simulink library "tqr"  (R2021b)
settings: Solver=VariableStepAuto  StartTime=0.0  StopTime=10.0  RelTol=1e-3
undefined symbols (not defined in the file or in its folder): ATQR_AltRDCActiveFEDUInc_X_pct, ATQR_AltRDCActiveFEDUInc_Y_enum, ATQR_AltRDCActiveFEDUTs_X_pct, ATQR_AltRDCActiveFEDUTs_Y_enum, ATQR_AltRDCActiveREDUInc_X_pct, ATQR_AltRDCActiveREDUInc_Y_enum, ATQR_AltRDCActiveREDUTs_X_pct, ATQR_AltRDCActiveREDUTs_Y_enum, ATQR_CreepFEDUTqIncSR_X_rpm, ATQR_CreepFEDUTqIncSR_Y_Nm, ATQR_CreepFEDUTs_X_rpm, ATQR_CreepFEDUTs_Y_Nm, ATQR_EcoTqFrIncGain_X_Nm, ATQR_EcoTqFrIncGain_Y_pct, ATQR_EcoTqRrIncGain_X_Nm, ATQR_EcoTqRrIncGain_Y_pct, ATQR_EL1FEDUTqDecSR_Y_Nm, ATQR_EL1FEDUTqIncSR_X_rpm, ATQR_EL1FEDUTqIncSR_Y_pct, ATQR_EL1FEDUTs_X_rpm, ATQR_EL1FEDUTs_Y_Nm, ATQR_EL1REDUTqDecSR_Y_Nm, ATQR_EL1REDUTs_Y_Nm, ATQR_FEDUEL1RegenTs_X_rpm, ATQR_FEDUTIPOutTs_X_rpm, ATQR_FrNegRateLimitIncN_X_rpm, ATQR_FrNegRateLimitIncN_Y_Nm, ATQR_FrPosRateLimitIncN_X_rpm, ATQR_FrPosRateLimitIncN_Y_Nm, ATQR_FShaftSpdTqLimCoe_X_rpm, ATQR_FTimerTqLimCoe_X_s, ATQR_FTqZeroTransUpBoundN_X_rpm, ATQR_NL1FEDUTqDecSR_Y_Nm, ATQR_NL1FEDUTqIncSR_X_rpm, ATQR_NL1FEDUTqIncSR_Y_pct, ATQR_NL1FEDUTs_X_rpm, ATQR_NL1FEDUTs_Y_Nm, ATQR_NL1REDUTqDecSR_Y_Nm, ATQR_NL1REDUTs_Y_Nm, ATQR_NormalTqFrIncGain_X_Nm, ATQR_NormalTqFrIncGain_Y_pct, ATQR_NormalTqRrIncGain_X_Nm, ATQR_NormalTqRrIncGain_Y_pct, ATQR_RrNegRateLimitIncN_X_rpm, ATQR_RrNegRateLimitIncN_Y_Nm, ATQR_RrPosRateLimitIncN_X_rpm, ATQR_RrPosRateLimitIncN_Y_Nm, ATQR_RShaftSpdTqLimCoe_X_rpm, ATQR_RTimerTqLimCoe_X_s, ATQR_SL1FEDUTqDecSR_Y_Nm, ATQR_SL1FEDUTqIncSR_X_rpm, ATQR_SL1FEDUTqIncSR_Y_pct, ATQR_SL1FEDUTs_X_rpm, ATQR_SL1FEDUTs_Y_Nm, ATQR_SL1REDUTqDecSR_Y_Nm, ATQR_SL1REDUTs_Y_Nm, ATQR_SportTqFrIncGain_X_Nm, ATQR_SportTqFrIncGain_Y_pct, ATQR_SportTqRrIncGain_X_Nm, ATQR_SportTqRrIncGain_Y_pct ... (+269)
libraries: hcu_lib x15, simulink x13, $bdroot x3
(part 1 of 9)
settings Model: Creator=13615  LastModifiedBy=FVT23118
settings SolverCC: AlgebraicLoopSolver=TrustRegion
settings DataIOCC: SaveFormat=Array  SignalLoggingSaveFormat=ModelDataLogs  ReturnWorkspaceOutputs=off
settings OptimizationCC: BlockReduction=off  BooleanDataType=off
settings DebuggingCC: SaveWithParameterizedLinksMsg=none  UnderspecifiedInitializationDetection=Classic  MergeDetectMultiDrivingBlocksExec=none  SignalResolutionControl=TryResolveAllWithWarning  SFMachineParentedDataDiag=warning
settings HardwareCC: TargetUnknown=on
settings ModelReferenceCC: PropagateSignalLabelsOutOfModel=off
settings ConfigComp: CovMetricSettings=dw  CovSaveCumulativeToWorkspaceVar=on  CovSaveSingleToWorkspaceVar=on

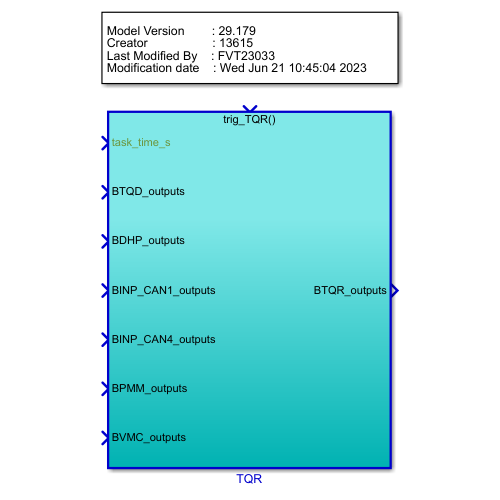
[thumbnail: Simulink's stored preview of the top-level diagram]
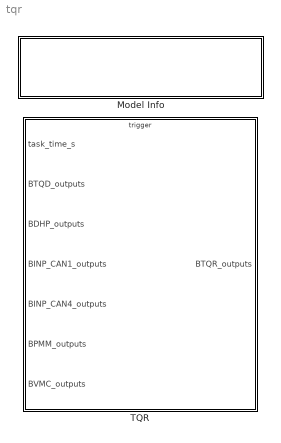
== system tqr ==
  Model Info : Subsystem  LoadFcn=slcm LoadBlock;  InitFcn=slcm('UpdateAllCMBlocksInThisModelInit')  mask(CMBlock){InitialSaveTempField=, InitialBlockCM=None, BlockCM=None, Frame=on, SaveTempField=, DisplayStringWithTags=|, MaskDisplayString=Model Version        : 29.417\nCreator                   : 13615\nLast Modified By    : FVT23118\nModification date    : Thu Aug 29 10:52:14 2024, HorizontalTextAlignment=Left, LeftAlignmentValue=0.02, SourceBlockDiagram=tqr, TagMaxNumber=20, CMTag1=, CMTag2=, CMTag3=, CMTag4=, CMTag5=, CMTag6=, CMTag7=, CMTag8=, CMTag9=, CMTag10=, CMTag11=, CMTag12=, CMTag13=, CMTag14=, CMTag15=, CMTag16=, CMTag17=, CMTag18=, CMTag19=, CMTag20=}
      mask DisplayStringWithTags=|
      | Model Version        : %<ModelVersion>
      | Creator                   : %<Creator>
      | Last Modified By    : %<LastModifiedBy>
      | Modification date    : %<LastModificationDate>
      mask help: This block allows revision control information to be displayed within the model.
      settings: CopyFcn=slcm CopyBlock;  DeleteFcn=slcm Cancel;  PostSaveFcn=slcm('UpdateAllCMBlocksInThisModel')  NameChangeFcn=slcm Rename;  OpenFcn=slcm
      mask Display: text(str2num(LeftAlignmentValue), 0.5, MaskDisplayString, 'HorizontalAlignment', HorizontalTextAlignment)
  TQR : Subsystem  TreatAsAtomicUnit=on
      settings: RTWSystemCode=Nonreusable function  RTWFcnNameOpts=Use subsystem name  RTWFileNameOpts=Use subsystem name

== system tqr/Model Info ==
  EmptySubsystem : Subsystem

== system tqr/TQR ==
  task_time_s : Inport
  BTQD_outputs : Inport  Port=2  OutDataTypeStr=Bus: BTQD_outputs
  BDHP_outputs : Inport  Port=3  OutDataTypeStr=Bus: BDHP_outputs
  BINP_CAN1_outputs : Inport  Port=4  OutDataTypeStr=Bus: BINP_CAN1_outputs
  BINP_CAN4_outputs : Inport  Port=5  OutDataTypeStr=Bus: BINP_CAN4_outputs
  BPMM_outputs : Inport  Port=6  OutDataTypeStr=Bus: BPMM_outputs
  BVMC_outputs : Inport  Port=7  OutDataTypeStr=Bus: BVMC_outputs
  trig_TQR : TriggerPort  TriggerType=function-call  VariantControl=(inherit)
  Bus Creator : BusCreator  Inputs=9
  Bus Selector : BusSelector  OutputSignals=VINP_VehSpeed_kph,VINP_FrPTCSActive_flg,VINP_RrPTCSActive_flg,VINP_ADASForceIdle_flg,VINP_FrRBCActive_flg,VINP_RrRBCActive_flg,VINP_FrntAxlTrqReqBrk_Nm,VINP_RearAxlTrqReqBrk_Nm,VINP_FrntAxlTrqReqDrv_Nm,VINP_RearAxlTrqReqDrv_Nm,VINP_BrkSwSta_flg,VINP_GRADE_Deg,VINP_ACCVehHoldReq_flg
  Bus Selector1 : BusSelector  OutputSignals=VTQD_GearActualPosn_enum,VTQD_TqSourceFr_enum,VTQD_TqSourceRr_enum,VTQD_TqTargetShaftSpd_rpm,VTQD_EVDriveMode_enum,VTQD_EVDriveModeValid_flg,VTQD_AfterAvailableTqDemRr_Nm,VTQD_AfterAvailableTqDemFr_Nm,VTQD_RollRegenEnable_flg,VTQD_LimpHomeAct_flg,VTQD_LoSpdBrkCtrl_flg,VTQD_PreLoadHold_flg,VTQD_PreLoadPreEn_flg,VTQD_CreepPrLoadEnable_flg,VTQD_RDCActive_enum,VTQD_RegenTqLimitEn_flg,VTQD_PedAccTqEn_flg,VTQD_RegenMode_enum,VTQD_FrEDUAvailBrkRgnTq_Nm,VTQD_RrEDUAvailBrkRgnTq_Nm,VTQD_VehActSpd_kph
  Bus Selector2 : BusSelector  OutputSignals=VDHP_ActAPSPosn_pct
  Bus Selector3 : BusSelector  OutputSignals=VPMM_DrivetrainSelect_enum
  Bus Selector5 : BusSelector  OutputSignals=VVMC_ACCPedalOvrd_flg,VVMC_CCPedalOvrd_flg,VVMC_ADASActive_flg,VVMC_ActMaxSlideRate_pct,VVMC_EstSlope_Deg
  Determine Torque Request : Subsystem
  Terminator : Terminator
  BTQR_outputs : Outport  OutDataTypeStr=Bus: BTQR_outputs
  wires:
  Determine Torque Request/1(VTQR_FrTMTqReq_Nm) -> Bus Creator/1
  Bus Creator/1 -> BTQR_outputs/1  "BTQR_outputs"
  BTQD_outputs/1 -> Bus Selector1/1
  task_time_s/1 -> Determine Torque Request/1(task_time_s)  "task_time_s"
  Determine Torque Request/2(VTQR_FEDUTMSpdReq_rpm) -> Bus Creator/2
  Bus Selector1/1 -> Determine Torque Request/2(VTQD_GearActualPosn_enum)  "<VTQD_GearActualPosn_enum>"
  Bus Selector1/2 -> Determine Torque Request/3(VTQD_TqSourceFr_enum)  "<VTQD_TqSourceFr_enum>"
  Bus Selector1/4 -> Determine Torque Request/5(VTQD_TqTargetShaftSpd_rpm)  "<VTQD_TqTargetShaftSpd_rpm>"
  Determine Torque Request/3(VTQR_RrTMTqReq_Nm) -> Bus Creator/3
  Determine Torque Request/4(VTQR_REDUTMSpdReq_rpm) -> Bus Creator/4
  Bus Selector1/5 -> Determine Torque Request/6(<VTQD_EVDriveMode_enum>)  "<VTQD_EVDriveMode_enum>"
  Bus Selector1/7 -> Determine Torque Request/8(<VTQD_AfterAvailableTqDemRr_Nm>)  "<VTQD_AfterAvailableTqDemRr_Nm>"
  Bus Selector1/8 -> Determine Torque Request/9(<VTQD_AfterAvailableTqDemFr_Nm>)  "<VTQD_AfterAvailableTqDemFr_Nm>"
  Bus Selector1/9 -> Determine Torque Request/10(VTQD_RollRegenEnable_flg)  "<VTQD_RollRegenEnable_flg>"
  BINP_CAN1_outputs/1 -> Bus Selector/1
  Bus Selector/1 -> Determine Torque Request/25(VINP_VehSpeed_kph)  "<VINP_VehSpeed_kph>"
  Bus Selector1/10 -> Determine Torque Request/11(VTQD_LimpHomeAct_flg)  "<VTQD_LimpHomeAct_flg>"
  Bus Selector1/6 -> Determine Torque Request/7(VTQD_EVDriveModeValid_flg)  "<VTQD_EVDriveModeValid_flg>"
  BDHP_outputs/1 -> Bus Selector2/1
  Bus Selector2/1 -> Determine Torque Request/24(VDHP_ActAPSPosn_pct)  "<VDHP_ActAPSPosn_pct>"
  BPMM_outputs/1 -> Bus Selector3/1
  Bus Selector3/1 -> Determine Torque Request/23(VPMM_DriveTrainSelect_enum)  "<VPMM_DrivetrainSelect_enum>"
  Bus Selector1/3 -> Determine Torque Request/4(VTQD_TqSourceRr_enum)  "<VTQD_TqSourceRr_enum>"
  Bus Selector/4 -> Determine Torque Request/28(VINP_ADASForceIdle_flg)  "<VINP_ADASForceIdle_flg>"
  Bus Selector/2 -> Determine Torque Request/26(VINP_FrPTCSActive_flg)  "<VINP_FrPTCSActive_flg>"
  Bus Selector/3 -> Determine Torque Request/27(VINP_RrPTCSActive_flg)  "<VINP_RrPTCSActive_flg>"
  Bus Selector/5 -> Determine Torque Request/29(VINP_FrRBCActive_flg)  "<VINP_FrRBCActive_flg>"
  Bus Selector/6 -> Determine Torque Request/30(VINP_RrRBCActive_flg)  "<VINP_RrRBCActive_flg>"
  BINP_CAN4_outputs/1 -> Terminator/1
  Determine Torque Request/6(VTQR_ActualREDUWhlTqReq_Nm) -> Bus Creator/6
  Determine Torque Request/5(VTQR_ActualFEDUWhlTqReq_Nm) -> Bus Creator/5
  Bus Selector1/11 -> Determine Torque Request/12(VTQD_LoSpdBrkCtrl_flg)  "<VTQD_LoSpdBrkCtrl_flg>"
  BVMC_outputs/1 -> Bus Selector5/1
  Bus Selector5/1 -> Determine Torque Request/38(VVMC_ACCPedalOvrd_flg)  "<VVMC_ACCPedalOvrd_flg>"
  Bus Selector/7 -> Determine Torque Request/31(VINP_FrntAxlTrqReqBrk_Nm)  "<VINP_FrntAxlTrqReqBrk_Nm>"
  Bus Selector/8 -> Determine Torque Request/32(VINP_RearAxlTrqReqBrk_Nm)  "<VINP_RearAxlTrqReqBrk_Nm>"
  Determine Torque Request/7(VTQR_NoABSFEDUWhlTqReq_Nm) -> Bus Creator/7
  Determine Torque Request/8(VTQR_NoABSREDUWhlTqReq_Nm) -> Bus Creator/8
  Bus Selector1/12 -> Determine Torque Request/13(VTQD_PreLoadHold_flg)  "<VTQD_PreLoadHold_flg>"
  Bus Selector1/13 -> Determine Torque Request/14(VTQD_PreLoadPreEn_flg)  "<VTQD_PreLoadPreEn_flg>"
  Bus Selector5/2 -> Determine Torque Request/39(VVMC_CCPedalOvrd_flg)  "<VVMC_CCPedalOvrd_flg>"
  Bus Selector5/3 -> Determine Torque Request/40(VVMC_ADASActive_flg)  "<VVMC_ADASActive_flg>"
  Bus Selector1/14 -> Determine Torque Request/15(VTQD_CreepPrLoadEnable_flg)  "<VTQD_CreepPrLoadEnable_flg>"
  Bus Selector1/15 -> Determine Torque Request/16(VTQD_RDCActive_enum)  "<VTQD_RDCActive_enum>"
  Bus Selector/9 -> Determine Torque Request/33(VINP_FrntAxlTrqReqDrv_Nm)  "<VINP_FrntAxlTrqReqDrv_Nm>"
  Bus Selector/10 -> Determine Torque Request/34(VINP_RearAxlTrqReqDrv_Nm)  "<VINP_RearAxlTrqReqDrv_Nm>"
  Bus Selector5/4 -> Determine Torque Request/41(VVMC_ActMaxSlideRate_pct)  "<VVMC_ActMaxSlideRate_pct>"
  Bus Selector1/16 -> Determine Torque Request/17(VTQD_RegenTqLimitEn_flg)  "<VTQD_RegenTqLimitEn_flg>"
  Bus Selector1/17 -> Determine Torque Request/18(VTQD_PedAccTqEn_flg)  "<VTQD_PedAccTqEn_flg>"
  Bus Selector1/19 -> Determine Torque Request/20(VTQD_FrEDUAvailBrkRgnTq_Nm)  "<VTQD_FrEDUAvailBrkRgnTq_Nm>"
  Bus Selector1/20 -> Determine Torque Request/21(VTQD_RrEDUAvailBrkRgnTq_Nm)  "<VTQD_RrEDUAvailBrkRgnTq_Nm>"
  Bus Selector1/18 -> Determine Torque Request/19(VTQD_RegenMode_enum)  "<VTQD_RegenMode_enum>"
  Determine Torque Request/9(VTQR_ACCHoldPdovrdInc_flg) -> Bus Creator/9
  Bus Selector/11 -> Determine Torque Request/35(VINP_BrkSwSta_flg)  "<VINP_BrkSwSta_flg>"
  Bus Selector/12 -> Determine Torque Request/36(VINP_GRADE_deg)  "<VINP_GRADE_Deg>"
  Bus Selector/13 -> Determine Torque Request/37(VINP_ACCVehHoldReq_flg)  "<VINP_ACCVehHoldReq_flg>"
  Bus Selector1/21 -> Determine Torque Request/22(VTQD_VehActSpd_kph)  "<VTQD_VehActSpd_kph>"
  Bus Selector5/5 -> Determine Torque Request/42(VVMC_EstSlope_Deg)  "<VVMC_EstSlope_Deg>"

== system tqr/Model Info/EmptySubsystem ==

== system tqr/TQR/Determine Torque Request ==
  task_time_s : Inport
  VTQD_GearActualPosn_enum : Inport  Port=2
  VTQD_TqSourceFr_enum : Inport  Port=3
  VTQD_TqSourceRr_enum : Inport  Port=4
  VTQD_TqTargetShaftSpd_rpm : Inport  Port=5
  <VTQD_EVDriveMode_enum> : Inport  Port=6
  VTQD_EVDriveModeValid_flg : Inport  Port=7
  <VTQD_AfterAvailableTqDemRr_Nm> : Inport  Port=8
  <VTQD_AfterAvailableTqDemFr_Nm> : Inport  Port=9
  VTQD_RollRegenEnable_flg : Inport  Port=10
  VTQD_LimpHomeAct_flg : Inport  Port=11
  VTQD_LoSpdBrkCtrl_flg : Inport  Port=12
  VTQD_PreLoadHold_flg : Inport  Port=13
  VTQD_PreLoadPreEn_flg : Inport  Port=14
  VTQD_CreepPrLoadEnable_flg : Inport  Port=15
  VTQD_RDCActive_enum : Inport  Port=16
  VTQD_RegenTqLimitEn_flg : Inport  Port=17
  VTQD_PedAccTqEn_flg : Inport  Port=18
  VTQD_RegenMode_enum : Inport  Port=19
  VTQD_FrEDUAvailBrkRgnTq_Nm : Inport  Port=20
  VTQD_RrEDUAvailBrkRgnTq_Nm : Inport  Port=21
  VTQD_VehActSpd_kph : Inport  Port=22
  VPMM_DriveTrainSelect_enum : Inport  Port=23
  VDHP_ActAPSPosn_pct : Inport  Port=24
  VINP_VehSpeed_kph : Inport  Port=25
  VINP_FrPTCSActive_flg : Inport  Port=26
  VINP_RrPTCSActive_flg : Inport  Port=27
  VINP_ADASForceIdle_flg : Inport  Port=28
  VINP_FrRBCActive_flg : Inport  Port=29
  VINP_RrRBCActive_flg : Inport  Port=30
  VINP_FrntAxlTrqReqBrk_Nm : Inport  Port=31
  VINP_RearAxlTrqReqBrk_Nm : Inport  Port=32
  VINP_FrntAxlTrqReqDrv_Nm : Inport  Port=33
  VINP_RearAxlTrqReqDrv_Nm : Inport  Port=34
  VINP_BrkSwSta_flg : Inport  Port=35
  VINP_GRADE_deg : Inport  Port=36
  VINP_ACCVehHoldReq_flg : Inport  Port=37
  VVMC_ACCPedalOvrd_flg : Inport  Port=38
  VVMC_CCPedalOvrd_flg : Inport  Port=39
  VVMC_ADASActive_flg : Inport  Port=40
  VVMC_ActMaxSlideRate_pct : Inport  Port=41
  VVMC_EstSlope_Deg : Inport  Port=42
  Cast To Boolean : DataTypeConversion  OutDataTypeStr=boolean
  Constant : Constant  Value=ZERO_FLOAT  OutDataTypeStr=single
  Constant1 : Constant  Value=ZERO_FLOAT  OutDataTypeStr=single
  Data Type Conversion{,1..7} (8 alike) : DataTypeConversion
  TorqueArbitrament : Subsystem
  VTQR_FrTMTqReq_Nm : Outport
  VTQR_FEDUTMSpdReq_rpm : Outport  Port=2
  VTQR_RrTMTqReq_Nm : Outport  Port=3
  VTQR_REDUTMSpdReq_rpm : Outport  Port=4
  VTQR_ActualFEDUWhlTqReq_Nm : Outport  Port=5
  VTQR_ActualREDUWhlTqReq_Nm : Outport  Port=6
  VTQR_NoABSFEDUWhlTqReq_Nm : Outport  Port=7
  VTQR_NoABSREDUWhlTqReq_Nm : Outport  Port=8
  VTQR_ACCHoldPdovrdInc_flg : Outport  Port=9
  wires:
  TorqueArbitrament/1(VTQR_FrTMTqReq_Nm) -> Data Type Conversion/1
  Constant/1 -> Data Type Conversion1/1
  task_time_s/1 -> TorqueArbitrament/1(task_time_s)
  VTQD_GearActualPosn_enum/1 -> TorqueArbitrament/4(VTQD_GearActualPosn_enum)
  VTQD_TqSourceFr_enum/1 -> TorqueArbitrament/5(VTQD_TqSourceFr_enum)
  Data Type Conversion/1 -> VTQR_FrTMTqReq_Nm/1  "VTQR_FrTMTqReq_Nm"
  Data Type Conversion1/1 -> VTQR_FEDUTMSpdReq_rpm/1  "VTQR_FEDUTMSpdReq_rpm"
  VTQD_TqTargetShaftSpd_rpm/1 -> TorqueArbitrament/3(VTQD_TqTargetShaftSpd_rpm)
  VDHP_ActAPSPosn_pct/1 -> TorqueArbitrament/2(VDHP_ActAPSPosn_pct)
  TorqueArbitrament/2(VTQR_RrTMTqReq_Nm) -> Data Type Conversion2/1
  Data Type Conversion2/1 -> VTQR_RrTMTqReq_Nm/1  "VTQR_RrTMTqReq_Nm"
  Data Type Conversion3/1 -> VTQR_REDUTMSpdReq_rpm/1  "VTQR_REDUTMSpdReq_rpm"
  Constant1/1 -> Data Type Conversion3/1
  <VTQD_EVDriveMode_enum>/1 -> TorqueArbitrament/7(VTQD_EVDriveMode_enum)
  <VTQD_AfterAvailableTqDemRr_Nm>/1 -> TorqueArbitrament/9(VTQD_AfterAvailableTqDemRr_Nm)
  <VTQD_AfterAvailableTqDemFr_Nm>/1 -> TorqueArbitrament/10(VTQD_AfterAvailableTqDemFr_Nm)
  VTQD_RollRegenEnable_flg/1 -> TorqueArbitrament/11(VTQD_RollRegenEnable_flg)
  VINP_VehSpeed_kph/1 -> TorqueArbitrament/12(VINP_VehSpeed_kph)
  VPMM_DriveTrainSelect_enum/1 -> TorqueArbitrament/13(VPMM_DriveTrainSelect_enum)
  VTQD_LimpHomeAct_flg/1 -> TorqueArbitrament/14(VTQD_LimpHomeAct_flg)
  VTQD_EVDriveModeValid_flg/1 -> TorqueArbitrament/8(VTQD_EVDriveModeValid_flg)
  VTQD_TqSourceRr_enum/1 -> TorqueArbitrament/6(VTQD_TqSourceRr_enum)
  VINP_FrPTCSActive_flg/1 -> TorqueArbitrament/15(VINP_FrPTCSActive_flg)
  VINP_RrPTCSActive_flg/1 -> TorqueArbitrament/16(VINP_RrPTCSActive_flg)
  VINP_ADASForceIdle_flg/1 -> TorqueArbitrament/17(VINP_ADASForceIdle_flg)
  VINP_FrRBCActive_flg/1 -> TorqueArbitrament/18(VINP_FrRBCActive_flg)
  VINP_RrRBCActive_flg/1 -> TorqueArbitrament/19(VINP_RrRBCActive_flg)
  TorqueArbitrament/3(VTQR_ActualFEDUWhlTqReq_Nm) -> Data Type Conversion4/1
  TorqueArbitrament/4(VTQR_ActualREDUWhlTqReq_Nm) -> Data Type Conversion5/1
  Data Type Conversion4/1 -> VTQR_ActualFEDUWhlTqReq_Nm/1  "VTQR_ActualFEDUWhlTqReq_Nm"
  Data Type Conversion5/1 -> VTQR_ActualREDUWhlTqReq_Nm/1  "VTQR_ActualREDUWhlTqReq_Nm"
  VTQD_LoSpdBrkCtrl_flg/1 -> TorqueArbitrament/21(VTQD_LoSpdBrkCtrl_flg)
  VTQD_RDCActive_enum/1 -> TorqueArbitrament/22(VTQD_RDCActive_enum)
  VINP_FrntAxlTrqReqBrk_Nm/1 -> TorqueArbitrament/23(VINP_FrntAxlTrqReqBrk_Nm)
  VINP_RearAxlTrqReqBrk_Nm/1 -> TorqueArbitrament/24(VINP_RearAxlTrqReqBrk_Nm)
  VVMC_ACCPedalOvrd_flg/1 -> TorqueArbitrament/25(VVMC_ACCPedalOvrd_flg)
  VVMC_CCPedalOvrd_flg/1 -> TorqueArbitrament/26(VVMC_CCPedalOvrd_flg)
  Data Type Conversion6/1 -> VTQR_NoABSFEDUWhlTqReq_Nm/1  "VTQR_NoABSFEDUWhlTqReq_Nm"
  TorqueArbitrament/6(VTQR_NoABSREDUWhlTqReq_Nm) -> Data Type Conversion7/1
  TorqueArbitrament/5(VTQR_NoABSFEDUWhlTqReq_Nm) -> Data Type Conversion6/1
  VTQD_PreLoadHold_flg/1 -> TorqueArbitrament/27(VTQD_PreLoadHold_flg)
  VTQD_PreLoadPreEn_flg/1 -> TorqueArbitrament/28(VTQD_PreLoadPreEn_flg)
  VVMC_ADASActive_flg/1 -> TorqueArbitrament/29(VVMC_ADASActive_flg)
  VTQD_CreepPrLoadEnable_flg/1 -> TorqueArbitrament/30(VTQD_CreepPrLoadEnable_flg)
  VINP_FrntAxlTrqReqDrv_Nm/1 -> TorqueArbitrament/32(VINP_FrntAxlTrqReqDrv_Nm)
  VINP_RearAxlTrqReqDrv_Nm/1 -> TorqueArbitrament/33(VINP_RearAxlTrqReqDrv_Nm)
  Data Type Conversion7/1 -> VTQR_NoABSREDUWhlTqReq_Nm/1  "VTQR_NoABSREDUWhlTqReq_Nm"
  VVMC_ActMaxSlideRate_pct/1 -> TorqueArbitrament/31(VVMC_ActMaxSlideRate_pct)
  VTQD_RegenTqLimitEn_flg/1 -> TorqueArbitrament/34(VTQD_RegenTqLimitEn_flg)
  VTQD_PedAccTqEn_flg/1 -> TorqueArbitrament/35(VTQD_PedAccTqEn_flg)
  VTQD_FrEDUAvailBrkRgnTq_Nm/1 -> TorqueArbitrament/36(VTQD_FrEDUAvailBrkRgnTq_Nm)
  VTQD_RrEDUAvailBrkRgnTq_Nm/1 -> TorqueArbitrament/37(VTQD_RrEDUAvailBrkRgnTq_Nm)
  VTQD_RegenMode_enum/1 -> TorqueArbitrament/20(VTQD_RegenMode_enum)
  Cast To Boolean/1 -> VTQR_ACCHoldPdovrdInc_flg/1  "VTQR_ACCHoldPdovrdInc_flg"
  TorqueArbitrament/7(VTQR_ACCHoldPdovrdInc_flg) -> Cast To Boolean/1
  VINP_BrkSwSta_flg/1 -> TorqueArbitrament/38(VINP_BrkSwSta_flg)
  VINP_GRADE_deg/1 -> TorqueArbitrament/39(VINP_GRADE_deg)
  VTQD_VehActSpd_kph/1 -> TorqueArbitrament/40(VTQD_VehActSpd_kph)
  VINP_ACCVehHoldReq_flg/1 -> TorqueArbitrament/41(VINP_ACCVehHoldReq_flg)
  VVMC_EstSlope_Deg/1 -> TorqueArbitrament/42(VVMC_EstSlope_Deg)

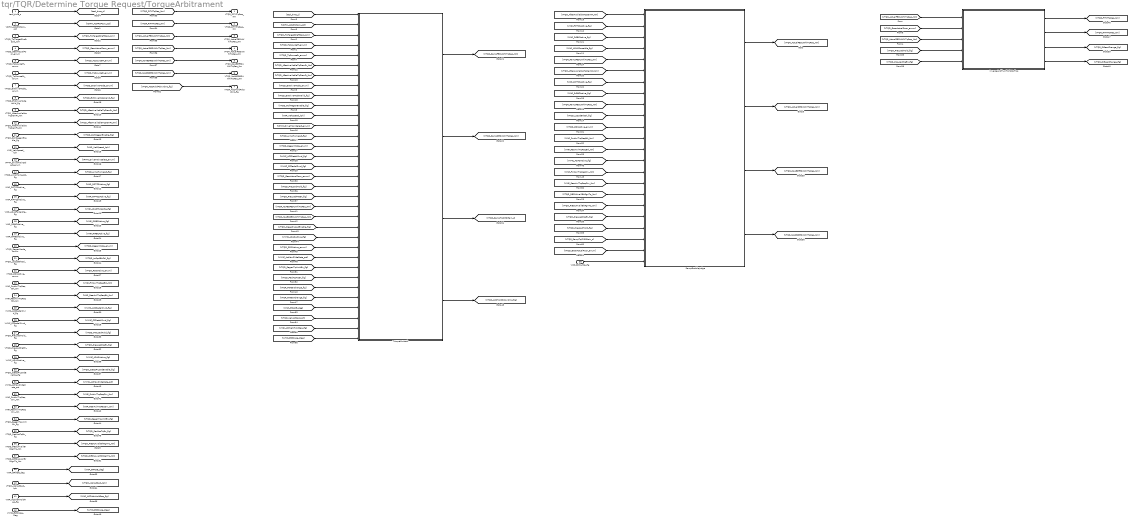
== system tqr/TQR/Determine Torque Request/TorqueArbitrament ==
  task_time_s : Inport
  VDHP_ActAPSPosn_pct : Inport  Port=2
  VTQD_TqTargetShaftSpd_rpm : Inport  Port=3
  VTQD_GearActualPosn_enum : Inport  Port=4
  VTQD_TqSourceFr_enum : Inport  Port=5
  VTQD_TqSourceRr_enum : Inport  Port=6
  VTQD_EVDriveMode_enum : Inport  Port=7
  VTQD_EVDriveModeValid_flg : Inport  Port=8
  VTQD_AfterAvailableTqDemRr_Nm : Inport  Port=9
  VTQD_AfterAvailableTqDemFr_Nm : Inport  Port=10
  VTQD_RollRegenEnable_flg : Inport  Port=11
  VINP_VehSpeed_kph : Inport  Port=12
  VPMM_DriveTrainSelect_enum : Inport  Port=13
  VTQD_LimpHomeAct_flg : Inport  Port=14
  VINP_FrPTCSActive_flg : Inport  Port=15
  VINP_RrPTCSActive_flg : Inport  Port=16
  VINP_ADASForceIdle_flg : Inport  Port=17
  VINP_FrRBCActive_flg : Inport  Port=18
  VINP_RrRBCActive_flg : Inport  Port=19
  VTQD_RegenMode_enum : Inport  Port=20
  VTQD_LoSpdBrkCtrl_flg : Inport  Port=21
  VTQD_RDCActive_enum : Inport  Port=22
  VINP_FrntAxlTrqReqBrk_Nm : Inport  Port=23
  VINP_RearAxlTrqReqBrk_Nm : Inport  Port=24
  VVMC_ACCPedalOvrd_flg : Inport  Port=25
  VVMC_CCPedalOvrd_flg : Inport  Port=26
  VTQD_PreLoadHold_flg : Inport  Port=27
  VTQD_PreLoadPreEn_flg : Inport  Port=28
  VVMC_ADASActive_flg : Inport  Port=29
  VTQD_CreepPrLoadEnable_flg : Inport  Port=30
  VVMC_ActMaxSlideRate_pct : Inport  Port=31
  VINP_FrntAxlTrqReqDrv_Nm : Inport  Port=32
  VINP_RearAxlTrqReqDrv_Nm : Inport  Port=33
  VTQD_RegenTqLimitEn_flg : Inport  Port=34
  VTQD_PedAccTqEn_flg : Inport  Port=35
  VTQD_FrEDUAvailBrkRgnTq_Nm : Inport  Port=36
  VTQD_RrEDUAvailBrkRgnTq_Nm : Inport  Port=37
  VINP_BrkSwSta_flg : Inport  Port=38
  VINP_GRADE_deg : Inport  Port=39
  VTQD_VehActSpd_kph : Inport  Port=40
  VINP_ACCVehHoldReq_flg : Inport  Port=41
  VVMC_EstSlope_Deg : Inport  Port=42
  InverseAndTurnToMotorToq : Subsystem
  RampEnableJudge : Subsystem
  TorqueSmooth : Subsystem
  VTQR_FrTMTqReq_Nm : Outport
  VTQR_RrTMTqReq_Nm : Outport  Port=2
  VTQR_ActualFEDUWhlTqReq_Nm : Outport  Port=3
  VTQR_ActualREDUWhlTqReq_Nm : Outport  Port=4
  VTQR_NoABSFEDUWhlTqReq_Nm : Outport  Port=5
  VTQR_NoABSREDUWhlTqReq_Nm : Outport  Port=6
  VTQR_ACCHoldPdovrdInc_flg : Outport  Port=7
  wires:
  task_time_s/1 -> [task_time_s]
  [task_time_s] -> TorqueSmooth/1(task_time_s)
  VTQD_GearActualPosn_enum/1 -> [VTQD_GearActualPosn_enum]
  [VTQD_GearActualPosn_enum] -> InverseAndTurnToMotorToq/2(VTQD_GearActualPosn_enum)
  VTQD_TqTargetShaftSpd_rpm/1 -> [VTQD_TqTargetShaftSpd_rpm]
  VTQD_TqSourceFr_enum/1 -> [VTQD_TqSourceFr_enum]
  [VTQD_TqSourceFr_enum] -> TorqueSmooth/4(VTQD_TqSourceFr_enum)
  [VTQD_TqTargetShaftSpd_rpm] -> TorqueSmooth/3(VTQD_TqTargetShaftSpd_rpm)
  VDHP_ActAPSPosn_pct/1 -> [VDHP_ActAPSPosn_pct]
  [VDHP_ActAPSPosn_pct] -> TorqueSmooth/2(VDHP_ActAPSPosn_pct)
  [VTQR_ActualFEDUWhlTqReq_Nm] -> InverseAndTurnToMotorToq/1(VTQR_ActualWhlTqReq_Nm)  "VTQR_ActualFEDUWhlTqReq_Nm"
  [VTQR_ActualREDUWhlTqReq_Nm] -> InverseAndTurnToMotorToq/3(VTQR_ActualREDUWhlTqReq_Nm)  "VTQR_ActualREDUWhlTqReq_Nm"
  VTQD_EVDriveMode_enum/1 -> [VTQD_EVDriveMode_enum]
  VTQD_AfterAvailableTqDemRr_Nm/1 -> [VTQD_AfterAvailableTqDemRr_Nm]
  VTQD_AfterAvailableTqDemFr_Nm/1 -> [VTQD_AfterAvailableTqDemFr_Nm]
  [VTQD_AfterAvailableTqDemFr_Nm] -> TorqueSmooth/7(VTQD_AfterAvailableTqDemFr_Nm)
  [VTQD_AfterAvailableTqDemRr_Nm] -> TorqueSmooth/6(VTQD_AfterAvailableTqDemRr_Nm)
  [VTQD_EVDriveMode_enum] -> TorqueSmooth/8(VTQD_EVDriveMode_enum)
  VTQD_RollRegenEnable_flg/1 -> [VTQD_RollRegenEnable_flg]
  [VTQD_RollRegenEnable_flg] -> TorqueSmooth/10(VTQD_RollRegenEnable_flg)
  VINP_VehSpeed_kph/1 -> [VINP_VehSpeed_kph]
  [VINP_VehSpeed_kph] -> TorqueSmooth/11(VINP_VehSpeed_kph)
  VPMM_DriveTrainSelect_enum/1 -> [VPMM_DriveTrainSelect_enum]
  [VPMM_DriveTrainSelect_enum] -> TorqueSmooth/12(VPMM_DriveTrainSelect_enum)
  VTQD_LimpHomeAct_flg/1 -> [VTQD_LimpHomeAct_flg]
  [VTQD_LimpHomeAct_flg] -> TorqueSmooth/13(VTQD_LimpHomeAct_flg)
  VTQD_EVDriveModeValid_flg/1 -> [VTQD_EVDriveModeValid_flg]
  [VTQD_EVDriveModeValid_flg] -> TorqueSmooth/9(VTQD_EVDriveModeValid_flg)
  VTQD_TqSourceRr_enum/1 -> [VTQD_TqSourceRr_enum]
  [VTQD_TqSourceRr_enum] -> TorqueSmooth/5(VTQD_TqSourceRr_enum)
  VINP_FrPTCSActive_flg/1 -> [VINP_FrPTCSActive_flg]
  VINP_RrPTCSActive_flg/1 -> [VINP_RrPTCSActive_flg]
  VINP_ADASForceIdle_flg/1 -> [VINP_ADASForceIdle_flg]
  [VINP_FrPTCSActive_flg] -> RampEnableJudge/2(VINP_FrPTCSActive_flg)
  [VINP_ADASForceIdle_flg] -> RampEnableJudge/4(VINP_ADASForceIdle_flg)
  [VINP_RrPTCSActive_flg] -> RampEnableJudge/7(VINP_RrPTCSActive_flg)
  RampEnableJudge/1(VTQR_ActualFEDUWhlTqReq_Nm) -> [VTQR_ActualFEDUWhlTqReq_Nm]
  RampEnableJudge/2(VTQR_ActualREDUWhlTqReq_Nm) -> [VTQR_ActualREDUWhlTqReq_Nm]
  [VTQR_RampFEDUWhlTqReq_Nm] -> RampEnableJudge/5(VTQR_RampFEDUWhlTqReq_Nm)
  TorqueSmooth/1(VTQR_RampFEDUWhlTqReq_Nm) -> [VTQR_RampFEDUWhlTqReq_Nm]
  TorqueSmooth/2(VTQR_RampREDUWhlTqReq_Nm) -> [VTQR_RampREDUWhlTqReq_Nm]
  [VTQR_RampREDUWhlTqReq_Nm] -> RampEnableJudge/9(VTQR_RampREDUWhlTqReq_Nm)
  VINP_FrRBCActive_flg/1 -> [VINP_FrRBCActive_flg]
  VINP_RrRBCActive_flg/1 -> [VINP_RrRBCActive_flg]
  [VINP_FrRBCActive_flg] -> RampEnableJudge/3(VINP_FrRBCActive_flg)
  [VINP_RrRBCActive_flg] -> RampEnableJudge/8(VINP_RrRBCActive_flg)
  VTQD_LoSpdBrkCtrl_flg/1 -> [VTQD_LoSpdBrkCtrl_flg]
  [VTQD_LoSpdBrkCtrl_flg] -> RampEnableJudge/10(VTQD_LoSpdBrkCtrl_flg)
  VTQD_RDCActive_enum/1 -> [VTQD_RDCActive_enum]
  VINP_FrntAxlTrqReqBrk_Nm/1 -> [VINP_FrntAxlTrqReqBrk_Nm]
  VINP_RearAxlTrqReqBrk_Nm/1 -> [VINP_RearAxlTrqReqBrk_Nm]
  VVMC_ACCPedalOvrd_flg/1 -> [VVMC_ACCPedalOvrd_flg]
  VVMC_CCPedalOvrd_flg/1 -> [VVMC_CCPedalOvrd_flg]
  [VVMC_ACCPedalOvrd_flg] -> TorqueSmooth/15(VVMC_ACCPedalOvrd_flg)
  [VVMC_CCPedalOvrd_flg] -> TorqueSmooth/16(VVMC_CCPedalOvrd_flg)
  [VTQD_GearActualPosn_enum] -> TorqueSmooth/17(VTQD_GearActualPosn_enum)
  [VTQD_RDCActive_enum] -> RampEnableJudge/11(VTQD_RDCActive_enum)
  [VINP_FrntAxlTrqReqBrk_Nm] -> RampEnableJudge/12(VINP_FrntAxlTrqReqBrk_Nm)
  [VINP_RearAxlTrqReqBrk_Nm] -> RampEnableJudge/13(VINP_RearAxlTrqReqBrk_Nm)
  RampEnableJudge/3(VTQR_NoABSFEDUWhlTqReq_Nm) -> [VTQR_NoABSFEDUWhlTqReq_Nm]
  VTQD_PreLoadPreEn_flg/1 -> [VTQD_PreLoadPreEn_flg]
  VTQD_PreLoadHold_flg/1 -> [VTQD_PreLoadHold_flg]
  [VTQD_PreLoadHold_flg] -> TorqueSmooth/18(VTQD_PreLoadHold_flg)
  [VTQD_PreLoadPreEn_flg] -> TorqueSmooth/19(VTQD_PreLoadPreEn_flg)
  [VTQD_PreLoadHold_flg] -> InverseAndTurnToMotorToq/4(VTQD_PreLoadHold_flg)
  [VTQD_PreLoadPreEn_flg] -> InverseAndTurnToMotorToq/5(VTQD_PreLoadPreEn_flg)
  [VTQR_NoABSFEDUWhlTqReq_Nm] -> TorqueSmooth/20(VTQR_NoABSFEDUWhlTqReq_Nm)
  [VTQR_NoABSREDUWhlTqReq_Nm] -> TorqueSmooth/21(VTQR_NoABSREDUWhlTqReq_Nm)
  VTQD_CreepPrLoadEnable_flg/1 -> [VTQD_CreepPrLoadEnable_flg]
  [VTQD_CreepPrLoadEnable_flg] -> TorqueSmooth/22(VTQD_CreepPrLoadEnable_flg)
  VVMC_ADASActive_flg/1 -> [VVMC_ADASActive_flg]
  [VVMC_ADASActive_flg] -> TorqueSmooth/23(VVMC_ADASActive_flg)
  [VTQD_RDCActive_enum] -> TorqueSmooth/24(VTQD_RDCActive_enum)
  [VVMC_ADASActive_flg] -> RampEnableJudge/14(VVMC_ADASActive_flg)
  [VTQD_AfterAvailableTqDemFr_Nm] -> RampEnableJudge/1(VTQD_AfterAvailableTqDemFr_Nm)
  [VTQD_AfterAvailableTqDemRr_Nm] -> RampEnableJudge/6(VTQD_AfterAvailableTqDemRr_Nm)
  VINP_RearAxlTrqReqDrv_Nm/1 -> [VINP_RearAxlTrqReqDrv_Nm]
  VINP_FrntAxlTrqReqDrv_Nm/1 -> [VINP_FrntAxlTrqReqDrv_Nm]
  [VINP_FrntAxlTrqReqDrv_Nm] -> RampEnableJudge/15(VINP_FrntAxlTrqReqDrv_Nm)
  [VINP_RearAxlTrqReqDrv_Nm] -> RampEnableJudge/16(VINP_RearAxlTrqReqDrv_Nm)
  VTQD_PedAccTqEn_flg/1 -> [VTQD_PedAccTqEn_flg]
  VTQD_RegenTqLimitEn_flg/1 -> [VTQD_RegenTqLimitEn_flg]
  VVMC_ActMaxSlideRate_pct/1 -> [VVMC_ActMaxSlideRate_pct]
  [VVMC_ActMaxSlideRate_pct] -> TorqueSmooth/25(VVMC_ActMaxSlideRate_pct)
  [VTQD_RegenTqLimitEn_flg] -> TorqueSmooth/26(VTQD_RegenTqLimitEn_flg)
  [VTQD_PedAccTqEn_flg] -> TorqueSmooth/27(VTQD_PedAccTqEn_flg)
  RampEnableJudge/4(VTQR_NoABSREDUWhlTqReq_Nm) -> [VTQR_NoABSREDUWhlTqReq_Nm]
  VTQD_FrEDUAvailBrkRgnTq_Nm/1 -> [VTQD_FrEDUAvailBrkRgnTq_Nm]
  VTQD_RrEDUAvailBrkRgnTq_Nm/1 -> [VTQD_RrEDUAvailBrkRgnTq_Nm]
  [VTQD_FrEDUAvailBrkRgnTq_Nm] -> RampEnableJudge/17(VTQD_FrEDUAvailBrkRgnTq_Nm)
  [VTQD_RrEDUAvailBrkRgnTq_Nm] -> RampEnableJudge/18(VTQD_RrEDUAvailBrkRgnTq_Nm)
  [VTQR_FrGearChange_flg] -> TorqueSmooth/28(VTQR_FrGearChange_flg)
  [VTQR_RrGearChange_flg] -> TorqueSmooth/29(VTQR_RrGearChange_flg)
  [VTQD_RegenMode_enum] -> TorqueSmooth/14(VTQD_RegenMode_enum)
  VTQD_RegenMode_enum/1 -> [VTQD_RegenMode_enum]
  InverseAndTurnToMotorToq/4(VTQR_RrGearChange_flg) -> [VTQR_RrGearChange_flg]
  InverseAndTurnToMotorToq/3(VTQR_FrGearChange_flg) -> [VTQR_FrGearChange_flg]
  InverseAndTurnToMotorToq/1(VTQR_FrTMTqReq_Nm) -> [VTQR_FrTMTqReq_Nm]
  InverseAndTurnToMotorToq/2(VTQR_RrTMTqReq_Nm) -> [VTQR_RrTMTqReq_Nm]
  [VTQR_RrTMTqReq_Nm] -> VTQR_RrTMTqReq_Nm/1
  [VTQR_FrTMTqReq_Nm] -> VTQR_FrTMTqReq_Nm/1
  [VTQR_ActualFEDUWhlTqReq_Nm] -> VTQR_ActualFEDUWhlTqReq_Nm/1
  [VTQR_ActualREDUWhlTqReq_Nm] -> VTQR_ActualREDUWhlTqReq_Nm/1
  [VTQR_NoABSFEDUWhlTqReq_Nm] -> VTQR_NoABSFEDUWhlTqReq_Nm/1
  [VTQR_NoABSREDUWhlTqReq_Nm] -> VTQR_NoABSREDUWhlTqReq_Nm/1
  [VTQD_PreLoadPreEn_flg] -> RampEnableJudge/19(VTQD_PreLoadPreEn_flg)
  [VTQD_PreLoadHold_flg] -> RampEnableJudge/20(VTQD_PreLoadHold_flg)
  [VTQR_RampTqCMDGain_c] -> RampEnableJudge/21(VTQR_RampTqCMDGain_c)
  TorqueSmooth/3(VTQR_RampTqCMDGain_c) -> [VTQR_RampTqCMDGain_c]
  [VTQD_GearActualPosn_enum] -> RampEnableJudge/22(VTQD_GearActualPosn_enum)
  [VTQR_ACCHoldPdovrdInc_flg] -> VTQR_ACCHoldPdovrdInc_flg/1
  VTQD_VehActSpd_kph/1 -> [VTQD_VehActSpd_kph]
  VINP_GRADE_deg/1 -> [VINP_GRADE_deg]
  VINP_ACCVehHoldReq_flg/1 -> [VINP_ACCVehHoldReq_flg]
  VINP_BrkSwSta_flg/1 -> RampEnableJudge/23(VINP_BrkSwSta_flg)
  [VINP_GRADE_deg] -> TorqueSmooth/30(VINP_GRADE_deg)
  [VTQD_VehActSpd_kph] -> TorqueSmooth/31(VTQD_VehActSpd_kph)
  [VINP_ACCVehHoldReq_flg] -> TorqueSmooth/32(VINP_ACCVehHoldReq_flg)
  TorqueSmooth/4(VTQR_ACCHoldPdovrdInc_flg) -> [VTQR_ACCHoldPdovrdInc_flg]
  [VVMC_EstSlope_Deg] -> TorqueSmooth/33(VVMC_EstSlope_Deg)
  VVMC_EstSlope_Deg/1 -> [VVMC_EstSlope_Deg]

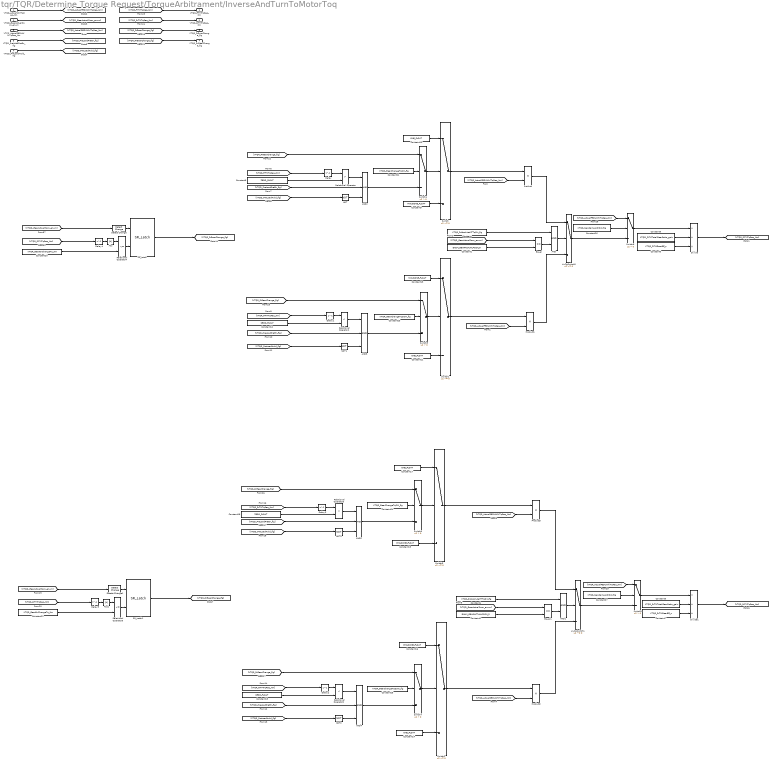
== system tqr/TQR/Determine Torque Request/TorqueArbitrament/InverseAndTurnToMotorToq ==
  VTQR_ActualWhlTqReq_Nm : Inport
  VTQD_GearActualPosn_enum : Inport  Port=2
  VTQR_ActualREDUWhlTqReq_Nm : Inport  Port=3
  VTQD_PreLoadHold_flg : Inport  Port=4
  VTQD_PreLoadPreEn_flg : Inport  Port=5
  AND : Logic  AllPortsSameDT=off  OutDataTypeStr=boolean
  AND1 : Logic  AllPortsSameDT=off  OutDataTypeStr=boolean
  AND{2..5} (4 alike) : Logic  Inputs=3  AllPortsSameDT=off  OutDataTypeStr=boolean
  Abs : Abs
  Abs1 : Abs
  Constant : Constant  Value=KTQR_FrAbsoluteMTTqDir_flg
  Constant1 : Constant  Value=ENUM_GEARACTUALPOSN_R
  Constant{10..11,14,17} (4 alike) : Constant  Value=ONE_FLOAT
  Constant{8,12,15,18} (4 alike) : Constant  Value=ZERO_FLOAT
  Constant{9,13,16,19} (4 alike) : Constant  Value=MINUSONE_FLOAT
  Constant2 : Constant  Value=ENUM_GEARACTUALPOSN_R
  Constant20 : Constant  Value=KTQR_GearEnChangeTq_Nm
  Constant21 : Constant  Value=KTQR_GearChangeTqSW_flg
  Constant22 : Constant  Value=KTQR_GearEnChangeTq_Nm
  Constant23 : Constant  Value=KTQR_GearChangeTqDSW_flg
  Constant24 : Constant  Value=KTQR_GearChangeTqSW_flg
  Constant25 : Constant  Value=KTQR_GearChangeTqDSW_flg
  Constant26 : Constant  Value=KTQR_NewRampArchSW_flg
  Constant27 : Constant  Value=KTQR_NewRampArchSW_flg
  Constant3 : Constant  Value=KTQD_RrTMTotalGearRatio_gain
  Constant4 : Constant  Value=KTQR_RrAbsoluteMTTqDir_flg
  Constant5 : Constant  Value=KTQD_FrTMTotalGearRatio_gain
  Constant6 : Constant  Value=KTQR_FrTMGearEff_c
  Constant7 : Constant  Value=KTQR_RrTMGearEff_c
  Delay{,1..5} (6 alike) : Delay  DelayLength=1
  Detect Change : simulink/Logic and Bit Operations/Detect Change  vinit=0  OutDataTypeStr=boolean
  Detect Change1 : simulink/Logic and Bit Operations/Detect Change  vinit=0  OutDataTypeStr=boolean
  Divide : Product  Inputs=*//
  Divide1 : Product  Inputs=*//
  Equal : RelationalOperator  Operator===  OutDataTypeStr=boolean  RndMeth=Simplest
  Equal1 : RelationalOperator  Operator===  OutDataTypeStr=boolean  RndMeth=Simplest
  LiuZgSwitch1 : Switch  Criteria=u2 ~= 0  Threshold=0.5
      settings: AttributesFormatString=<%<Criteria>>
  LiuZgSwitch8 : Switch  Criteria=u2 ~= 0  Threshold=0.5
      settings: AttributesFormatString=<%<Criteria>>
  NOT{,1..3} (4 alike) : Logic  Operator=NOT  AllPortsSameDT=off  OutDataTypeStr=boolean
  Product{,1..3} (4 alike) : Product
  Relational Operator : RelationalOperator  Operator=>  OutDataTypeStr=boolean  RndMeth=Simplest
  Relational Operator1 : RelationalOperator  Operator=<  OutDataTypeStr=boolean  RndMeth=Simplest
  Relational Operator2 : RelationalOperator  Operator=<  OutDataTypeStr=boolean  RndMeth=Simplest
  Relational Operator3 : RelationalOperator  Operator=>  OutDataTypeStr=boolean  RndMeth=Simplest
  Relational Operator4 : RelationalOperator  Operator=<=  OutDataTypeStr=boolean  RndMeth=Simplest
  Relational Operator5 : RelationalOperator  Operator=<=  OutDataTypeStr=boolean  RndMeth=Simplest
  SR_Latch : hcu_lib/Basic_Blocks/SR_Latch
  SR_Latch1 : hcu_lib/Basic_Blocks/SR_Latch
  Switch{,1..3} (4 alike) : Switch  Criteria=u2 ~= 0
  Switch{4..9} (6 alike) : Switch  Criteria=u2 > Threshold
  VTQR_FrTMTqReq_Nm : Outport
  VTQR_RrTMTqReq_Nm : Outport  Port=2
  VTQR_FrGearChange_flg : Outport  Port=3
  VTQR_RrGearChange_flg : Outport  Port=4
  wires:
  Relational Operator3/1 -> AND5/1
  Delay3/1 -> Relational Operator3/1
  [VTQR_RrTMTqReq_Nm] -> Delay2/1
  Constant6/1 -> Divide/3
  VTQD_PreLoadHold_flg/1 -> [VTQD_PreLoadHold_flg]
  NOT3/1 -> AND5/3
  Divide1/1 -> [VTQR_RrTMTqReq_Nm]  "VTQR_RrTMTqReq_Nm"
  [VTQD_PreLoadPreEn_flg] -> AND5/2
  Constant17/1 -> Switch3/1
  VTQD_PreLoadPreEn_flg/1 -> [VTQD_PreLoadPreEn_flg]
  [VTQD_PreLoadPreEn_flg] -> AND4/2
  Constant19/1 -> Switch3/3
  [VTQR_ActualREDUWhlTqReq_Nm] -> Product3/2
  [VTQR_ActualFEDUWhlTqReq_Nm] -> Product1/2
  Constant13/1 -> Switch1/1
  Constant18/1 -> Relational Operator3/2
  Product3/1 -> LiuZgSwitch1/1
  Divide/1 -> [VTQR_FrTMTqReq_Nm]  "VTQR_FrTMTqReq_Nm"
  VTQR_ActualWhlTqReq_Nm/1 -> [VTQR_ActualFEDUWhlTqReq_Nm]
  Constant/1 -> AND/1
  Constant15/1 -> Relational Operator2/2
  [VTQD_PreLoadHold_flg] -> NOT/1
  [VTQD_PreLoadHold_flg] -> NOT2/1
  Relational Operator2/1 -> AND4/1
  Constant12/1 -> Relational Operator1/2
  Switch2/1 -> Product2/1
  [VTQR_ActualREDUWhlTqReq_Nm] -> Product2/2
  [VTQR_FrTMTqReq_Nm] -> Delay/1
  NOT1/1 -> AND3/3
  Delay/1 -> Relational Operator/1
  Delay2/1 -> Relational Operator2/1
  Constant11/1 -> Switch1/3
  Product2/1 -> LiuZgSwitch1/3
  [VTQR_FrTMTqReq_Nm] -> Delay1/1
  NOT2/1 -> AND4/3
  [VTQD_PreLoadPreEn_flg] -> AND2/2
  Switch1/1 -> Product1/1
  Relational Operator1/1 -> AND3/1
  [VTQD_PreLoadPreEn_flg] -> AND3/2
  [VTQR_RrTMTqReq_Nm] -> Delay3/1
  [VTQD_PreLoadHold_flg] -> NOT1/1
  Constant9/1 -> Switch/3
  Delay1/1 -> Relational Operator1/1
  Constant14/1 -> Switch2/3
  Equal1/1 -> AND1/2
  Product/1 -> LiuZgSwitch8/1
  Constant4/1 -> AND1/1
  Switch3/1 -> Product3/1
  Equal/1 -> AND/2
  [VTQD_PreLoadHold_flg] -> NOT3/1
  Constant1/1 -> Equal/2
  Constant16/1 -> Switch2/1
  Constant8/1 -> Relational Operator/2
  Constant2/1 -> Equal1/2
  Product1/1 -> LiuZgSwitch8/3
  AND1/1 -> LiuZgSwitch1/2
  [VTQD_GearActualPosn_enum] -> Equal1/1
  VTQR_ActualREDUWhlTqReq_Nm/1 -> [VTQR_ActualREDUWhlTqReq_Nm]  "VTQR_ActualREDUWhlTqReq_Nm"
  Constant10/1 -> Switch/1
  Relational Operator/1 -> AND2/1
  NOT/1 -> AND2/3
  Constant5/1 -> Divide/2
  [VTQR_ActualFEDUWhlTqReq_Nm] -> Product/2
  Constant3/1 -> Divide1/2
  Constant7/1 -> Divide1/3
  AND/1 -> LiuZgSwitch8/2
  VTQD_GearActualPosn_enum/1 -> [VTQD_GearActualPosn_enum]
  [VTQD_GearActualPosn_enum] -> Equal/1
  Switch/1 -> Product/1
  SR_Latch/1 -> [VTQR_FrGearChange_flg]  "VTQR_FrGearChange_flg"
  Delay4/1 -> Abs/1
  [VTQR_RrTMTqReq_Nm] -> Delay5/1
  Abs/1 -> Relational Operator4/1
  Relational Operator5/1 -> SR_Latch1/2
  Detect Change1/1 -> SR_Latch1/1
  [VTQD_GearActualPosn_enum] -> Detect Change1/1
  Constant22/1 -> Relational Operator5/2
  Abs1/1 -> Relational Operator5/1
  Delay5/1 -> Abs1/1
  SR_Latch1/1 -> [VTQR_RrGearChange_flg]  "VTQR_RrGearChange_flg"
  Relational Operator4/1 -> SR_Latch/2
  [VTQD_GearActualPosn_enum] -> Detect Change/1
  [VTQR_FrTMTqReq_Nm] -> Delay4/1
  Constant20/1 -> Relational Operator4/2
  Detect Change/1 -> SR_Latch/1
  [VTQR_FrGearChange_flg] -> VTQR_FrGearChange_flg/1
  [VTQR_RrGearChange_flg] -> VTQR_RrGearChange_flg/1
  Switch4/1 -> Switch/2
  Constant21/1 -> Switch4/2
  [VTQR_FrGearChange_flg] -> Switch4/1
  AND2/1 -> Switch4/3
  [VTQR_FrTMTqReq_Nm] -> VTQR_FrTMTqReq_Nm/1
  [VTQR_RrTMTqReq_Nm] -> VTQR_RrTMTqReq_Nm/1
  Switch5/1 -> Switch1/2
  [VTQR_FrGearChange_flg] -> Switch5/1
  Constant23/1 -> Switch5/2
  AND3/1 -> Switch5/3
  [VTQR_RrGearChange_flg] -> Switch6/1
  Switch6/1 -> Switch3/2
  Constant24/1 -> Switch6/2
  AND5/1 -> Switch6/3
  Switch7/1 -> Switch2/2
  Constant25/1 -> Switch7/2
  [VTQR_RrGearChange_flg] -> Switch7/1
  AND4/1 -> Switch7/3
  LiuZgSwitch8/1 -> Switch8/3
  Switch8/1 -> Divide/1  "VTQR_InitFEDUWhlTqReq_Nm"
  Constant26/1 -> Switch8/2
  [VTQR_ActualFEDUWhlTqReq_Nm] -> Switch8/1
  [VTQR_ActualFEDUWhlTqReq_Nm] -> Switch9/1
  Constant27/1 -> Switch9/2
  LiuZgSwitch1/1 -> Switch9/3
  Switch9/1 -> Divide1/1  "VTQR_InitREDUWhlTqReq_Nm"

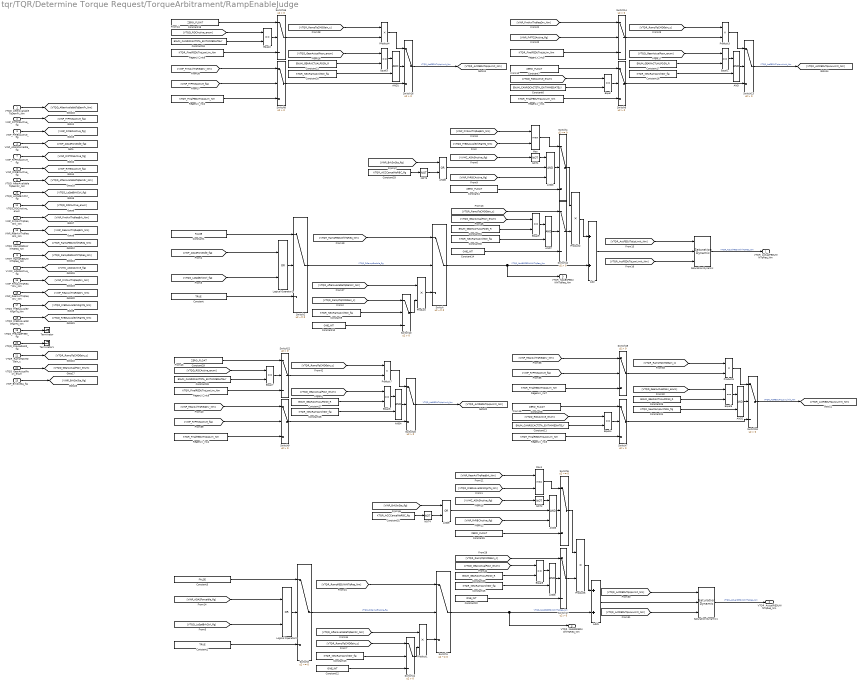
== system tqr/TQR/Determine Torque Request/TorqueArbitrament/RampEnableJudge ==
  VTQD_AfterAvailableTqDemFr_Nm : Inport
  VINP_FrPTCSActive_flg : Inport  Port=2
  VINP_FrRBCActive_flg : Inport  Port=3
  VINP_ADASForceIdle_flg : Inport  Port=4
  VTQR_RampFEDUWhlTqReq_Nm : Inport  Port=5
  VTQD_AfterAvailableTqDemRr_Nm : Inport  Port=6
  VINP_RrPTCSActive_flg : Inport  Port=7
  VINP_RrRBCActive_flg : Inport  Port=8
  VTQR_RampREDUWhlTqReq_Nm : Inport  Port=9
  VTQD_LoSpdBrkCtrl_flg : Inport  Port=10
  VTQD_RDCActive_enum : Inport  Port=11
  VINP_FrntAxlTrqReqBrk_Nm : Inport  Port=12
  VINP_RearAxlTrqReqBrk_Nm : Inport  Port=13
  VVMC_ADASActive_flg : Inport  Port=14
  VINP_FrntAxlTrqReqDrv_Nm : Inport  Port=15
  VINP_RearAxlTrqReqDrv_Nm : Inport  Port=16
  VTQD_FrEDUAvailBrkRgnTq_Nm : Inport  Port=17
  VTQD_RrEDUAvailBrkRgnTq_Nm : Inport  Port=18
  VTQD_PreLoadPreEn_flg : Inport  Port=19
  VTQD_PreLoadHold_flg : Inport  Port=20
  VTQR_RampTqCMDGain_c : Inport  Port=21
  VTQD_GearActualPosn_enum : Inport  Port=22
  VINP_BrkSwSta_flg : Inport  Port=23
  AND{,1..2,4,6..7} (6 alike) : Logic  AllPortsSameDT=off  OutDataTypeStr=boolean
  AND3 : Logic  Inputs=3  AllPortsSameDT=off  OutDataTypeStr=boolean
  AND5 : Logic  Inputs=3  AllPortsSameDT=off  OutDataTypeStr=boolean
  AND8 : Logic  Operator=OR  AllPortsSameDT=off  OutDataTypeStr=boolean
  AND9 : Logic  Operator=OR  AllPortsSameDT=off  OutDataTypeStr=boolean
  Add : Sum
  Add1 : Sum
  Constant : Constant  Value=TRUE
  Constant1 : Constant  Value=FALSE
  Constant{10,12,14,22} (4 alike) : Constant  Value=ONE_INT
  Constant{6,11,18,28} (4 alike) : Constant  Value=ENUM_CANRDCACTSTA_EXITIMMEDIATELY
  Constant{9,13,15..16,20,24,26,30} (8 alike) : Constant  Value=KTQR_NewRampArchSW_flg
  Constant{17,21,23,25,27,31} (6 alike) : Constant  Value=ENUM_GEARACTUALPOSN_R
  Constant{4..5,7..8,19,29} (6 alike) : Constant  Value=ZERO_FLOAT
  Constant2 : Constant  Value=TRUE
  Constant3 : Constant  Value=FALSE
  Constant32 : Constant  Value=KTQR_ACCCancelNoRBC_flg
  Constant33 : Constant  Value=KTQR_ACCCancelNoRBC_flg
  Equal{,1..9} (10 alike) : RelationalOperator  Operator===  OutDataTypeStr=boolean  RndMeth=Simplest
  Logical Operator1 : Logic  Operator=OR  AllPortsSameDT=off  OutDataTypeStr=boolean
  Logical Operator2 : Logic  Operator=OR  AllPortsSameDT=off  OutDataTypeStr=boolean
  Max : MinMax  Function=max  Inputs=2
  Max1 : MinMax  Function=max  Inputs=2
  NOT{1..4} (4 alike) : Logic  Operator=NOT  AllPortsSameDT=off  OutDataTypeStr=boolean
  Product{,1..7} (8 alike) : Product
  RegenLV_inc1 : Constant  Value=KTQR_FinalFEDUTrqLowLim_Nm  OutDataTypeStr=single
  RegenLV_inc2 : Constant  Value=KTQR_FinalFEDUTrqUpLim_Nm  OutDataTypeStr=single
  RegenLV_inc3 : Constant  Value=KTQR_FinalREDUTrqLowLim_Nm  OutDataTypeStr=single
  RegenLV_inc4 : Constant  Value=KTQR_FinalREDUTrqUpLim_Nm  OutDataTypeStr=single
  RegenLV_inc5 : Constant  Value=KTQR_FinalFEDUTrqUpLim_Nm  OutDataTypeStr=single
  RegenLV_inc6 : Constant  Value=KTQR_FinalFEDUTrqLowLim_Nm  OutDataTypeStr=single
  RegenLV_inc7 : Constant  Value=KTQR_FinalREDUTrqUpLim_Nm  OutDataTypeStr=single
  RegenLV_inc8 : Constant  Value=KTQR_FinalREDUTrqLowLim_Nm  OutDataTypeStr=single
  Saturation Dynamic : simulink/Discontinuities/Saturation Dynamic  OutMin=[]  OutMax=[]  OutDataTypeStr=Inherit: Same as second input  OutDataType=fixdt(1, 16)  OutScaling=2^-10  DoSatur=off
  Saturation Dynamic1 : simulink/Discontinuities/Saturation Dynamic  OutMin=[]  OutMax=[]  OutDataTypeStr=Inherit: Same as second input  OutDataType=fixdt(1, 16)  OutScaling=2^-10  DoSatur=off
  Switch{,1..5} (6 alike) : Switch  Criteria=u2 ~= 0
  Switch{6..21} (16 alike) : Switch  Criteria=u2 > Threshold
  Terminator : Terminator
  Terminator1 : Terminator
  VTQR_ActualFEDUWhlTqReq_Nm : Outport
  VTQR_ActualREDUWhlTqReq_Nm : Outport  Port=2
  VTQR_NoABSFEDUWhlTqReq_Nm : Outport  Port=3
  VTQR_NoABSREDUWhlTqReq_Nm : Outport  Port=4
  wires:
  VINP_ADASForceIdle_flg/1 -> [VINP_ADASForceIdle_flg]
  VINP_FrPTCSActive_flg/1 -> [VINP_FrPTCSActive_flg]
  VINP_RrPTCSActive_flg/1 -> [VINP_RrPTCSActive_flg]
  VINP_FrRBCActive_flg/1 -> [VINP_FrRBCActive_flg]
  VINP_RrRBCActive_flg/1 -> [VINP_RrRBCActive_flg]
  VTQD_LoSpdBrkCtrl_flg/1 -> [VTQD_LoSpdBrkCtrl_flg]
  VTQD_RDCActive_enum/1 -> [VTQD_RDCActive_enum]
  VINP_FrntAxlTrqReqBrk_Nm/1 -> [VINP_FrntAxlTrqReqBrk_Nm]
  VINP_RearAxlTrqReqBrk_Nm/1 -> [VINP_RearAxlTrqReqBrk_Nm]
  VTQR_RampFEDUWhlTqReq_Nm/1 -> [VTQR_RampFEDUWhlTqReq_Nm]
  VTQR_RampREDUWhlTqReq_Nm/1 -> [VTQR_RampREDUWhlTqReq_Nm]
  VVMC_ADASActive_flg/1 -> [VVMC_ADASActive_flg]
  VTQD_AfterAvailableTqDemFr_Nm/1 -> [VTQD_AfterAvailableTqDemFr_Nm]
  VTQD_AfterAvailableTqDemRr_Nm/1 -> [VTQD_AfterAvailableTqDemRr_Nm]
  VINP_RearAxlTrqReqDrv_Nm/1 -> [VINP_RearAxlTrqReqDrv_Nm]
  VINP_FrntAxlTrqReqDrv_Nm/1 -> [VINP_FrntAxlTrqReqDrv_Nm]
  Constant7/1 -> Switch6/1
  [VINP_ADASForceIdle_flg] -> Logical Operator1/1
  [VINP_FrPTCSActive_flg] -> Switch8/2
  Constant2/1 -> Switch3/3
  Constant6/1 -> Equal/2
  RegenLV_inc2/1 -> Switch8/3
  Constant1/1 -> Switch2/1
  [VTQR_RampREDUWhlTqReq_Nm] -> Switch1/1
  Switch2/1 -> Switch/2  "VTQR_FrRampEnable_flg"
  Constant3/1 -> Switch3/1
  Saturation Dynamic/1 -> VTQR_ActualFEDUWhlTqReq_Nm/1  "VTQR_ActualFEDUWhlTqReq_Nm"
  Logical Operator1/1 -> Switch2/2
  RegenLV_inc4/1 -> Switch9/3
  Constant8/1 -> Switch7/1
  Equal4/1 -> Switch7/2
  Constant11/1 -> Equal4/2
  [VTQD_RDCActive_enum] -> Equal/1
  [VINP_FrntAxlTrqReqDrv_Nm] -> Switch8/1
  Constant5/1 -> Switch5/3
  Equal/1 -> Switch6/2
  Switch3/1 -> Switch1/2  "VTQR_RrRampEnable_flg"
  [VTQD_RDCActive_enum] -> Equal4/1
  NOT1/1 -> AND3/1
  Logical Operator2/1 -> Switch3/2
  Add1/1 -> Saturation Dynamic1/2
  [VINP_RearAxlTrqReqDrv_Nm] -> Switch9/1
  Saturation Dynamic1/1 -> VTQR_ActualREDUWhlTqReq_Nm/1  "VTQR_ActualREDUWhlTqReq_Nm"
  [VTQR_RampFEDUWhlTqReq_Nm] -> Switch/1
  Add/1 -> Saturation Dynamic/2
  Constant/1 -> Switch2/3
  [VVMC_ADASActive_flg] -> NOT2/1
  NOT2/1 -> AND5/1
  AND3/1 -> Switch4/2
  AND5/1 -> Switch5/2
  [VVMC_ADASActive_flg] -> NOT1/1
  [VINP_RrRBCActive_flg] -> AND5/3
  Switch/1 -> VTQR_NoABSFEDUWhlTqReq_Nm/1, Add/2  "VTQR_NoABSFEDUWhlTqReq_Nm"
  Constant4/1 -> Switch4/3
  Switch1/1 -> Add1/2, VTQR_NoABSREDUWhlTqReq_Nm/1  "VTQR_NoABSREDUWhlTqReq_Nm"
  RegenLV_inc1/1 -> Switch6/3
  [VINP_RrPTCSActive_flg] -> Switch9/2
  [VINP_FrRBCActive_flg] -> AND3/3
  RegenLV_inc3/1 -> Switch7/3
  VTQD_FrEDUAvailBrkRgnTq_Nm/1 -> [VTQD_FrEDUAvailBrkRgnTq_Nm]
  VTQD_RrEDUAvailBrkRgnTq_Nm/1 -> [VTQD_RrEDUAvailBrkRgnTq_Nm]
  Max/1 -> Switch4/1
  [VTQD_FrEDUAvailBrkRgnTq_Nm] -> Max/2
  [VINP_FrntAxlTrqReqBrk_Nm] -> Max/1
  Max1/1 -> Switch5/1
  [VTQD_RrEDUAvailBrkRgnTq_Nm] -> Max1/2
  [VINP_RearAxlTrqReqBrk_Nm] -> Max1/1
  VTQD_PreLoadHold_flg/1 -> Terminator1/1
  VTQD_PreLoadPreEn_flg/1 -> Terminator/1
  [VINP_ADASForceIdle_flg] -> Logical Operator2/1
  [VTQD_LoSpdBrkCtrl_flg] -> Logical Operator1/2
  [VTQD_LoSpdBrkCtrl_flg] -> Logical Operator2/2
  VTQR_RampTqCMDGain_c/1 -> [VTQR_RampTqCMDGain_c]
  Product/1 -> Switch/3
  [VTQD_AfterAvailableTqDemFr_Nm] -> Product/1
  Switch10/1 -> Product/2
  [VTQR_RampTqCMDGain_c] -> Switch10/1
  Constant9/1 -> Switch10/2
  Constant10/1 -> Switch10/3
  Constant13/1 -> Switch11/2
  Switch11/1 -> Product1/2
  Constant12/1 -> Switch11/3
  Product1/1 -> Switch1/3
  [VTQD_AfterAvailableTqDemRr_Nm] -> Product1/1
  [VTQR_RampTqCMDGain_c] -> Switch11/1
  Constant14/1 -> Switch12/3
  [VTQR_RampTqCMDGain_c] -> Switch12/1
  Switch12/1 -> Product2/2
  Product2/1 -> Add/1
  Switch4/1 -> Product2/1
  [VTQR_ActFEDUTqLowLimit_Nm] -> Saturation Dynamic/3
  Switch6/1 -> Switch13/3
  Switch13/1 -> [VTQR_ActFEDUTqLowLimit_Nm]  "VTQR_ActFEDUTqLowLimit_Nm"
  AND/1 -> Switch13/2
  Constant16/1 -> AND/2
  VTQD_GearActualPosn_enum/1 -> [VTQD_GearActualPosn_enum]
  Equal1/1 -> AND/1
  [VTQD_GearActualPosn_enum] -> Equal1/1
  Constant17/1 -> Equal1/2
  [VINP_FrPTCSActive_flg] -> Switch14/2
  [VINP_FrntAxlTrqReqDrv_Nm] -> Switch14/1
  RegenLV_inc5/1 -> Switch14/3
  Product3/1 -> Switch13/1
  Switch14/1 -> Product3/2
  [VTQR_RampTqCMDGain_c] -> Product3/1
  Equal2/1 -> Switch15/2
  RegenLV_inc6/1 -> Switch15/3
  [VTQD_RDCActive_enum] -> Equal2/1
  Constant18/1 -> Equal2/2
  Constant19/1 -> Switch15/1
  [VTQR_RampTqCMDGain_c] -> Product4/1
  AND1/1 -> Switch16/2
  Equal3/1 -> AND1/1
  Constant21/1 -> Equal3/2
  Product4/1 -> Switch16/1
  Constant20/1 -> AND1/2
  [VTQD_GearActualPosn_enum] -> Equal3/1
  Switch15/1 -> Product4/2
  Switch8/1 -> Switch16/3
  Switch16/1 -> [VTQR_ActFEDUTqUpLimit_Nm]  "VTQR_ActFEDUTqUpLimit_Nm"
  [VTQR_RampTqCMDGain_c] -> Switch17/1
  Constant22/1 -> Switch17/3
  Switch5/1 -> Product5/1
  Product5/1 -> Add1/1
  [VTQR_ActREDUTqLowLimit_Nm] -> Saturation Dynamic1/3
  [VTQR_RampTqCMDGain_c] -> Product6/1
  AND2/1 -> Switch18/2
  Equal5/1 -> AND2/1
  Constant25/1 -> Equal5/2
  Product6/1 -> Switch18/1
  Constant24/1 -> AND2/2
  [VTQD_GearActualPosn_enum] -> Equal5/1
  Switch19/1 -> Product6/2
  Switch7/1 -> Switch18/3
  Switch18/1 -> [VTQR_ActREDUTqLowLimit_Nm]  "VTQR_ActREDUTqLowLimit_Nm"
  [VINP_RrPTCSActive_flg] -> Switch19/2
  [VINP_RearAxlTrqReqDrv_Nm] -> Switch19/1
  RegenLV_inc7/1 -> Switch19/3
  Product7/1 -> Switch20/1
  Constant27/1 -> Equal6/2
  [VTQD_GearActualPosn_enum] -> Equal6/1
  Equal6/1 -> AND4/1
  Constant26/1 -> AND4/2
  [VTQR_RampTqCMDGain_c] -> Product7/1
  Switch21/1 -> Product7/2
  AND4/1 -> Switch20/2
  Switch9/1 -> Switch20/3
  Switch20/1 -> [VTQR_ActREDUTqUpLimit_Nm]  "VTQR_ActREDUTqUpLimit_Nm"
  [VTQR_ActREDUTqUpLimit_Nm] -> Saturation Dynamic1/1
  [VTQR_ActFEDUTqUpLimit_Nm] -> Saturation Dynamic/1
  RegenLV_inc8/1 -> Switch21/3
  Constant29/1 -> Switch21/1
  Equal7/1 -> Switch21/2
  Constant28/1 -> Equal7/2
  [VTQD_RDCActive_enum] -> Equal7/1
  Switch17/1 -> Product5/2
  Equal8/1 -> AND6/1
  Constant23/1 -> Equal8/2
  Constant15/1 -> AND6/2
  [VTQD_GearActualPosn_enum] -> Equal8/1
  AND6/1 -> Switch17/2
  Constant30/1 -> AND7/2
  [VTQD_GearActualPosn_enum] -> Equal9/1
  Constant31/1 -> Equal9/2
  Equal9/1 -> AND7/1
  AND7/1 -> Switch12/2
  NOT3/1 -> AND8/2
  NOT4/1 -> AND9/2
  Constant32/1 -> NOT4/1
  [VINP_BrkSwSta_flg] -> AND9/1
  [VINP_BrkSwSta_flg] -> AND8/1
  Constant33/1 -> NOT3/1
  VINP_BrkSwSta_flg/1 -> [VINP_BrkSwSta_flg]
  AND8/1 -> AND3/2
  AND9/1 -> AND5/2
